simulink model "B2B_2x15kW_LCO_paralelo_y_serie"  (R2026b)
settings: Solver=ode5  StopTime=inf  EnableMultiTasking=on
StopFcn:
  | Modelo_Disable_B2B
undefined symbols (not defined in the file): ALPHA_DC, COS_RO, dataStateMachine, DiscIntNeverNeededParam, dq2abc, EN_G, getNormalizedOffset, I_MAX_G, INV_SIN_RO, KAW_CCG, KAW_DC, KI_CCG, KI_DC, KI_PLLG, KP_CCG, KP_DC, KP_PLLG, L12, LIMIT_SAG_DETECT, magnitude, MIN_VDC_READY, Ncount, NDELAY_SAG_DETECT, PORC_DC_STEADS, SAMPLES_SAG_DETECT, simDCcontCurrent1, simDCcontCurrent2, SN_G, Transformations_blocks, ts, Ts_al, TS_C, TS_PLL, UDC_min_al, UDC_Ref_al, VDC_REF, WN_G
libraries: simulink x15, TriPhaseDriveControl x13, powerlib_extras x2, model_hardware_PM15F80C_rev x2, TriphaseXenomaiTarget x1
(part 3 of 4)

== system B2B_2x15kW_LCO_paralelo_y_serie/VSC1 Controller2/Grid Side Measurements/D-LCO FLL/Sequence Detection/LCO_FLL_3_harm_alfa ==
  note: Para que no se valla a inf
  note: los regresamos
      | a la ganancia
      | original
  note: 1 sobre la ganancia
      | del interarmónico
      | 1/0.05 = 20
  v_in : Inport
  reset_LCO_FLL : Inport  Port=2
  Constant1 : Constant  Value=50
  Demux1 : Demux  Outputs=5
  Demux4 : Demux  Outputs=3
  Discrete-Time Integrator1 : DiscreteIntegrator  gainval=[1 1 1]  ExternalReset=either  InitialCondition=[1 1 10]  SampleTime=TS_PLL  ICPrevOutput=DiscIntNeverNeededParam  ICPrevScaledInput=DiscIntNeverNeededParam
  K gain : Constant  Value=0.1
  LCO_FLL_01 : MATLAB Function  TreatAsAtomicUnit=on
  Mux1 : Mux  Inputs=3
  Mux4 : Mux  Inputs=2
  Mux6 : Mux  Inputs=3
  Saturation2 : Saturate  UpperLimit=10000  LowerLimit=-10000
  Sinch 3 harm paralel : Scope
      settings: TimeSpan=0.1  ActiveDisplayYMinimum=-60  ActiveDisplayYMaximum=80  DataLoggingVariableName=LCO_FLL_graph3_paralelo
  Terminator3 : Terminator
  delta w : Scope
      settings: TimeSpan=20  ActiveDisplayYMinimum=-31  ActiveDisplayYMaximum=-24  DataLoggingVariableName=ScopeData4
  freq : Scope
      settings: TimeSpan=10  ActiveDisplayYMinimum=308  ActiveDisplayYMaximum=322  DataLoggingVariableName=w_LCO2_paralelo
  ki1 : Gain  Gain=2
  ki2 : Gain  Gain=1/(2*pi)
  ki3 : Gain  Gain=1/2
  ki4 : Gain  Gain=1/2
  v_out : Outport
  qv_out : Outport  Port=2
  tag scope: f_alfa_3=global
  wires:
  Discrete-Time Integrator1/1 -> Saturation2/1, Demux4/1
  Saturation2/1 -> Mux6/1
  v_in/1 -> ki1/1
  Constant1/1 -> Mux6/2  "A"
  Mux1/1 -> Discrete-Time Integrator1/1
  reset_LCO_FLL/1 -> Discrete-Time Integrator1/2
  Demux4/3 -> delta w/1, Terminator3/1  "x3 -  delta w"
  Demux4/1 -> ki3/1  "x1 - qv '"
  Demux4/2 -> Mux4/2, ki4/1  "x2 - v '"
  Demux1/1 -> LCO_FLL_01/1(x1)
  Mux6/1 -> Demux1/1
  Demux1/2 -> LCO_FLL_01/2(x2)
  Demux1/3 -> LCO_FLL_01/3(x3)
  Demux1/4 -> LCO_FLL_01/4(A)
  Demux1/5 -> LCO_FLL_01/5(v)
  LCO_FLL_01/1(x1p) -> Mux1/1
  LCO_FLL_01/2(x2p) -> Mux1/2
  LCO_FLL_01/3(x3p) -> Mux1/3
  LCO_FLL_01/4(w) -> ki2/1
  ki2/1 -> [f_alfa_3], freq/1
  Mux4/1 -> Sinch 3 harm paralel/1
  ki4/1 -> v_out/1
  ki3/1 -> qv_out/1
  ki1/1 -> Mux4/1, Mux6/3
  K gain/1 -> LCO_FLL_01/6(k)

== system B2B_2x15kW_LCO_paralelo_y_serie/VSC1 Controller2/Grid Side Measurements/D-LCO FLL/Sequence Detection/LCO_FLL_3_harm_alfa1 ==
  note: Para que no se valla a inf
  note: los regresamos
      | a la ganancia
      | original
  note: 1 sobre la ganancia
      | del interarmónico
      | 1/0.05 = 20
  v_in : Inport
  reset_LCO_FLL : Inport  Port=2
  Constant1 : Constant  Value=50
  Demux1 : Demux  Outputs=5
  Demux4 : Demux  Outputs=3
  Discrete-Time Integrator1 : DiscreteIntegrator  gainval=[1 1 1]  ExternalReset=either  InitialCondition=[1 1 10]  SampleTime=TS_PLL  ICPrevOutput=DiscIntNeverNeededParam  ICPrevScaledInput=DiscIntNeverNeededParam
  K gain : Constant  Value=0.1
  LCO_FLL_01 : MATLAB Function  TreatAsAtomicUnit=on
  Mux1 : Mux  Inputs=3
  Mux4 : Mux  Inputs=2
  Mux6 : Mux  Inputs=3
  Saturation2 : Saturate  UpperLimit=10000  LowerLimit=-10000
  Sinch 3 harm serie : Scope
      settings: TimeSpan=0.1  ActiveDisplayYMinimum=-60  ActiveDisplayYMaximum=80  DataLoggingVariableName=LCO_FLL_graph03_serie
  Terminator3 : Terminator
  delta w : Scope
      settings: TimeSpan=20  ActiveDisplayYMinimum=-31  ActiveDisplayYMaximum=-24  DataLoggingVariableName=ScopeData4
  freq alfa 3 : Scope
      settings: TimeSpan=10  ActiveDisplayYMinimum=529  ActiveDisplayYMaximum=536  DataLoggingVariableName=w_LCO2_serie
  ki1 : Gain  Gain=2
  ki2 : Gain  Gain=1/(2*pi)
  ki3 : Gain  Gain=1/2
  ki4 : Gain  Gain=1/2
  v_out : Outport
  qv_out : Outport  Port=2
  tag scope: f_alfa_3_serie=global
  wires:
  Discrete-Time Integrator1/1 -> Saturation2/1, Demux4/1
  Saturation2/1 -> Mux6/1
  v_in/1 -> ki1/1
  Constant1/1 -> Mux6/2  "A"
  Mux1/1 -> Discrete-Time Integrator1/1
  reset_LCO_FLL/1 -> Discrete-Time Integrator1/2
  Demux4/3 -> delta w/1, Terminator3/1  "x3 -  delta w"
  Demux4/1 -> ki3/1  "x1 - qv '"
  Demux4/2 -> Mux4/2, ki4/1  "x2 - v '"
  Demux1/1 -> LCO_FLL_01/1(x1)
  Mux6/1 -> Demux1/1
  Demux1/2 -> LCO_FLL_01/2(x2)
  Demux1/3 -> LCO_FLL_01/3(x3)
  Demux1/4 -> LCO_FLL_01/4(A)
  Demux1/5 -> LCO_FLL_01/5(v)
  LCO_FLL_01/1(x1p) -> Mux1/1
  LCO_FLL_01/2(x2p) -> Mux1/2
  LCO_FLL_01/3(x3p) -> Mux1/3
  LCO_FLL_01/4(w) -> ki2/1
  ki2/1 -> [f_alfa_3_serie], freq alfa 3/1
  ki1/1 -> Mux4/1, Mux6/3
  ki3/1 -> qv_out/1
  ki4/1 -> v_out/1
  Mux4/1 -> Sinch 3 harm serie/1
  K gain/1 -> LCO_FLL_01/6(k)

== system B2B_2x15kW_LCO_paralelo_y_serie/VSC1 Controller2/Grid Side Measurements/D-LCO FLL/Sequence Detection/LCO_FLL_4_harm_alfa ==
  note: Para que no se valla a inf
  note: los regresamos
      | a la ganancia
      | original
  note: 1 sobre la ganancia
      | del interarmónico
      | 1/0.05 = 20
  v_in : Inport
  reset_LCO_FLL : Inport  Port=2
  Constant1 : Constant  Value=150
  Demux1 : Demux  Outputs=5
  Demux4 : Demux  Outputs=3
  Discrete-Time Integrator1 : DiscreteIntegrator  gainval=[1 1 1]  ExternalReset=either  InitialCondition=[1 1 10]  SampleTime=TS_PLL  ICPrevOutput=DiscIntNeverNeededParam  ICPrevScaledInput=DiscIntNeverNeededParam
  K gain : Constant  Value=0.1
  LCO_FLL_01 : MATLAB Function  TreatAsAtomicUnit=on
  Mux1 : Mux  Inputs=3
  Mux4 : Mux  Inputs=2
  Mux6 : Mux  Inputs=3
  Saturation2 : Saturate  UpperLimit=500  LowerLimit=-500
  Sinch 4 harm paralel : Scope
      settings: TimeSpan=0.1  ActiveDisplayYMinimum=-300  ActiveDisplayYMaximum=300  DataLoggingVariableName=LCO_FLL_graph4_paralelo
  Terminator3 : Terminator
  delta w : Scope
      settings: TimeSpan=20  ActiveDisplayYMinimum=-31  ActiveDisplayYMaximum=-24  DataLoggingVariableName=ScopeData4
  freq : Scope
      settings: TimeSpan=10  ActiveDisplayYMinimum=308  ActiveDisplayYMaximum=322  DataLoggingVariableName=w_LCO3_paralelo
  ki1 : Gain  Gain=5
  ki2 : Gain  Gain=1/(2*pi)
  ki3 : Gain  Gain=1/5
  ki4 : Gain  Gain=1/5
  v_out : Outport
  qv_out : Outport  Port=2
  tag scope: f_alfa_4=global
  wires:
  LCO_FLL_01/4(w) -> ki2/1
  LCO_FLL_01/3(x3p) -> Mux1/3
  LCO_FLL_01/2(x2p) -> Mux1/2
  LCO_FLL_01/1(x1p) -> Mux1/1
  Demux1/5 -> LCO_FLL_01/5(v)
  Demux1/4 -> LCO_FLL_01/4(A)
  Demux1/3 -> LCO_FLL_01/3(x3)
  Demux1/2 -> LCO_FLL_01/2(x2)
  Mux6/1 -> Demux1/1
  Demux1/1 -> LCO_FLL_01/1(x1)
  Demux4/2 -> Mux4/2, ki4/1  "x2 - v '"
  Demux4/1 -> ki3/1  "x1 - qv '"
  Demux4/3 -> Terminator3/1, delta w/1  "x3 -  delta w"
  reset_LCO_FLL/1 -> Discrete-Time Integrator1/2
  Mux1/1 -> Discrete-Time Integrator1/1
  Constant1/1 -> Mux6/2  "A"
  v_in/1 -> ki1/1
  Saturation2/1 -> Mux6/1
  Discrete-Time Integrator1/1 -> Demux4/1, Saturation2/1
  ki2/1 -> [f_alfa_4], freq/1
  Mux4/1 -> Sinch 4 harm paralel/1
  ki3/1 -> qv_out/1
  ki4/1 -> v_out/1
  ki1/1 -> Mux4/1, Mux6/3
  K gain/1 -> LCO_FLL_01/6(k)

== system B2B_2x15kW_LCO_paralelo_y_serie/VSC1 Controller2/Grid Side Measurements/D-LCO FLL/Sequence Detection/LCO_FLL_4_harm_alfa1 ==
  note: Para que no se valla a inf
  note: los regresamos
      | a la ganancia
      | original
  note: 1 sobre la ganancia
      | del interarmónico
      | 1/0.05 = 20
  v_in : Inport
  reset_LCO_FLL : Inport  Port=2
  Constant1 : Constant  Value=150
  Demux1 : Demux  Outputs=5
  Demux4 : Demux  Outputs=3
  Discrete-Time Integrator1 : DiscreteIntegrator  gainval=[1 1 1]  ExternalReset=either  InitialCondition=[1 1 10]  SampleTime=TS_PLL  ICPrevOutput=DiscIntNeverNeededParam  ICPrevScaledInput=DiscIntNeverNeededParam
  K gain : Constant  Value=0.1
  LCO_FLL_01 : MATLAB Function  TreatAsAtomicUnit=on
  Mux1 : Mux  Inputs=3
  Mux4 : Mux  Inputs=2
  Mux6 : Mux  Inputs=3
  Saturation2 : Saturate  UpperLimit=5000  LowerLimit=-5000
  Sinch 4 harm serie : Scope
      settings: TimeSpan=0.1  ActiveDisplayYMinimum=-300  ActiveDisplayYMaximum=300  DataLoggingVariableName=LCO_FLL_graph04_serie
  Terminator3 : Terminator
  delta w : Scope
      settings: TimeSpan=20  ActiveDisplayYMinimum=-31  ActiveDisplayYMaximum=-24  DataLoggingVariableName=ScopeData4
  freq alfa 4 : Scope
      settings: TimeSpan=10  ActiveDisplayYMinimum=308  ActiveDisplayYMaximum=322  DataLoggingVariableName=w_LCO3_serie
  ki1 : Gain  Gain=5
  ki2 : Gain  Gain=1/(2*pi)
  ki3 : Gain  Gain=1/5
  ki4 : Gain  Gain=1/5
  v_out : Outport
  qv_out : Outport  Port=2
  tag scope: f_alfa_4_serie=global
  wires:
  LCO_FLL_01/4(w) -> ki2/1
  LCO_FLL_01/3(x3p) -> Mux1/3
  LCO_FLL_01/2(x2p) -> Mux1/2
  LCO_FLL_01/1(x1p) -> Mux1/1
  Demux1/5 -> LCO_FLL_01/5(v)
  Demux1/4 -> LCO_FLL_01/4(A)
  Demux1/3 -> LCO_FLL_01/3(x3)
  Demux1/2 -> LCO_FLL_01/2(x2)
  Mux6/1 -> Demux1/1
  Demux1/1 -> LCO_FLL_01/1(x1)
  Demux4/2 -> Mux4/2, ki4/1  "x2 - v '"
  Demux4/1 -> ki3/1  "x1 - qv '"
  Demux4/3 -> Terminator3/1, delta w/1  "x3 -  delta w"
  reset_LCO_FLL/1 -> Discrete-Time Integrator1/2
  Mux1/1 -> Discrete-Time Integrator1/1
  Constant1/1 -> Mux6/2  "A"
  v_in/1 -> ki1/1
  Saturation2/1 -> Mux6/1
  Discrete-Time Integrator1/1 -> Demux4/1, Saturation2/1
  ki2/1 -> [f_alfa_4_serie], freq alfa 4/1
  K gain/1 -> LCO_FLL_01/6(k)
  ki1/1 -> Mux4/1, Mux6/3
  ki4/1 -> v_out/1
  ki3/1 -> qv_out/1
  Mux4/1 -> Sinch 4 harm serie/1

== system B2B_2x15kW_LCO_paralelo_y_serie/VSC1 Controller2/Grid Side Measurements/D-LCO FLL/Sequence Detection/LCO_FLL_5_harm_alfa ==
  note: Para que no se valla a inf
  note: los regresamos
      | a la ganancia
      | original
  note: 1 sobre la ganancia
      | del interarmónico
      | 1/0.05 = 20
  v_in : Inport
  reset_LCO_FLL : Inport  Port=2
  Constant1 : Constant  Value=150
  Demux1 : Demux  Outputs=5
  Demux4 : Demux  Outputs=3
  Discrete-Time Integrator1 : DiscreteIntegrator  gainval=[1 1 1]  ExternalReset=either  InitialCondition=[1 1 10]  SampleTime=TS_PLL  ICPrevOutput=DiscIntNeverNeededParam  ICPrevScaledInput=DiscIntNeverNeededParam
  K gain : Constant  Value=0.1
  LCO_FLL_01 : MATLAB Function  TreatAsAtomicUnit=on
  Mux1 : Mux  Inputs=3
  Mux4 : Mux  Inputs=2
  Mux6 : Mux  Inputs=3
  Saturation2 : Saturate  UpperLimit=5000  LowerLimit=-5000
  Sinch 5 harm paralel : Scope
      settings: TimeSpan=0.1  ActiveDisplayYMinimum=-300  ActiveDisplayYMaximum=300  DataLoggingVariableName=LCO_FLL_graph5_paralelo
  Terminator3 : Terminator
  delta w : Scope
      settings: TimeSpan=20  ActiveDisplayYMinimum=-31  ActiveDisplayYMaximum=-24  DataLoggingVariableName=ScopeData4
  freq : Scope
      settings: TimeSpan=10  ActiveDisplayYMinimum=308  ActiveDisplayYMaximum=322  DataLoggingVariableName=w_LCO4_paralelo
  ki1 : Gain  Gain=5
  ki2 : Gain  Gain=1/(2*pi)
  ki3 : Gain  Gain=1/5
  ki4 : Gain  Gain=1/5
  v_out : Outport
  qv_out : Outport  Port=2
  tag scope: f_alfa_5=global
  wires:
  Discrete-Time Integrator1/1 -> Saturation2/1, Demux4/1
  Saturation2/1 -> Mux6/1
  v_in/1 -> ki1/1
  Constant1/1 -> Mux6/2  "A"
  Mux1/1 -> Discrete-Time Integrator1/1
  reset_LCO_FLL/1 -> Discrete-Time Integrator1/2
  Demux4/3 -> delta w/1, Terminator3/1  "x3 -  delta w"
  Demux4/1 -> ki3/1  "x1 - qv '"
  Demux4/2 -> Mux4/2, ki4/1  "x2 - v '"
  Demux1/1 -> LCO_FLL_01/1(x1)
  Mux6/1 -> Demux1/1
  Demux1/2 -> LCO_FLL_01/2(x2)
  Demux1/3 -> LCO_FLL_01/3(x3)
  Demux1/4 -> LCO_FLL_01/4(A)
  Demux1/5 -> LCO_FLL_01/5(v)
  LCO_FLL_01/1(x1p) -> Mux1/1
  LCO_FLL_01/2(x2p) -> Mux1/2
  LCO_FLL_01/3(x3p) -> Mux1/3
  LCO_FLL_01/4(w) -> ki2/1
  ki2/1 -> [f_alfa_5], freq/1
  Mux4/1 -> Sinch 5 harm paralel/1
  ki1/1 -> Mux4/1, Mux6/3
  K gain/1 -> LCO_FLL_01/6(k)
  ki3/1 -> qv_out/1
  ki4/1 -> v_out/1

== system B2B_2x15kW_LCO_paralelo_y_serie/VSC1 Controller2/Grid Side Measurements/D-LCO FLL/Sequence Detection/LCO_FLL_5_harm_alfa1 ==
  note: Para que no se valla a inf
  v_in : Inport
  reset_LCO_FLL : Inport  Port=2
  Constant1 : Constant  Value=158
  Demux1 : Demux  Outputs=5
  Demux4 : Demux  Outputs=3
  Discrete-Time Integrator1 : DiscreteIntegrator  gainval=[1 1 1]  ExternalReset=either  InitialCondition=[1 1 10]  SampleTime=TS_PLL  ICPrevOutput=DiscIntNeverNeededParam  ICPrevScaledInput=DiscIntNeverNeededParam
  K gain : Constant  Value=0.1
  LCO_FLL_01 : MATLAB Function  TreatAsAtomicUnit=on
  Mux1 : Mux  Inputs=3
  Mux6 : Mux  Inputs=3
  Saturation2 : Saturate  UpperLimit=5000  LowerLimit=-5000
  Terminator3 : Terminator
  delta w : Scope
      settings: TimeSpan=20  ActiveDisplayYMinimum=-31  ActiveDisplayYMaximum=-24  DataLoggingVariableName=ScopeData4
  freq alfa 5 : Scope
      settings: TimeSpan=10  ActiveDisplayYMinimum=308  ActiveDisplayYMaximum=322  DataLoggingVariableName=w_LCO4_serie
  ki2 : Gain  Gain=1/(2*pi)
  v_out : Outport
  qv_out : Outport  Port=2
  wires:
  Discrete-Time Integrator1/1 -> Saturation2/1, Demux4/1
  Saturation2/1 -> Mux6/1
  v_in/1 -> Mux6/3
  Constant1/1 -> Mux6/2  "A"
  Mux1/1 -> Discrete-Time Integrator1/1
  reset_LCO_FLL/1 -> Discrete-Time Integrator1/2
  Demux4/3 -> delta w/1, Terminator3/1  "x3 -  delta w"
  Demux4/1 -> qv_out/1  "x1 - qv '"
  Demux4/2 -> v_out/1  "x2 - v '"
  Demux1/1 -> LCO_FLL_01/1(x1)
  Mux6/1 -> Demux1/1
  Demux1/2 -> LCO_FLL_01/2(x2)
  Demux1/3 -> LCO_FLL_01/3(x3)
  Demux1/4 -> LCO_FLL_01/4(A)
  Demux1/5 -> LCO_FLL_01/5(v)
  LCO_FLL_01/1(x1p) -> Mux1/1
  LCO_FLL_01/2(x2p) -> Mux1/2
  LCO_FLL_01/3(x3p) -> Mux1/3
  LCO_FLL_01/4(w) -> ki2/1
  ki2/1 -> freq alfa 5/1
  K gain/1 -> LCO_FLL_01/6(k)

== system B2B_2x15kW_LCO_paralelo_y_serie/VSC1 Controller2/Grid Side Measurements/D-LCO FLL/Sequence Detection/LCO_FLL_main_ALFA ==
  note: Para que no se valla a inf
  note: 1 sobre la ganancia
      | del interarmónico
      | 1/0.05 = 20
  note: los regresamos
      | a la ganancia
      | original
  v_in : Inport
  reset_LCO_FLL : Inport  Port=2
  Constant1 : Constant  Value=158
  Demux1 : Demux  Outputs=5
  Demux4 : Demux  Outputs=3
  Discrete-Time Integrator1 : DiscreteIntegrator  gainval=[1 1 1]  ExternalReset=either  InitialCondition=[1 1 10]  SampleTime=TS_PLL  ICPrevOutput=DiscIntNeverNeededParam  ICPrevScaledInput=DiscIntNeverNeededParam
  K gain : Constant  Value=0.1
  LCO_FLL_01 : MATLAB Function  TreatAsAtomicUnit=on
  Mux1 : Mux  Inputs=3
  Mux4 : Mux  Inputs=2
  Mux6 : Mux  Inputs=3
  Saturation2 : Saturate  UpperLimit=500  LowerLimit=-500
  Sinch 1 harm paralel : Scope
      settings: TimeSpan=0.1  ActiveDisplayYMinimum=-200  ActiveDisplayYMaximum=200  DataLoggingVariableName=LCO_FLL_graph1_paralelo
  Terminator3 : Terminator
  delta w : Scope
      settings: TimeSpan=20  ActiveDisplayYMinimum=-31  ActiveDisplayYMaximum=-24  DataLoggingVariableName=ScopeData4
  freq : Scope
      settings: TimeSpan=10  ActiveDisplayYMinimum=308  ActiveDisplayYMaximum=322  DataLoggingVariableName=w_LCO
  ki1 : Gain
  ki2 : Gain  Gain=1/(2*pi)
  ki3 : Gain
  ki4 : Gain
  v_out : Outport
  qv_out : Outport  Port=2
  tag scope: f_alfa_1=global, w_alfa_LCO=global
  wires:
  Discrete-Time Integrator1/1 -> Saturation2/1, Demux4/1
  Saturation2/1 -> Mux6/1
  v_in/1 -> ki1/1
  Constant1/1 -> Mux6/2  "A"
  Mux1/1 -> Discrete-Time Integrator1/1
  reset_LCO_FLL/1 -> Discrete-Time Integrator1/2
  Demux4/3 -> delta w/1, Terminator3/1  "x3 -  delta w"
  Demux4/1 -> ki3/1  "x1 - qv '"
  Demux4/2 -> Mux4/2, ki4/1  "x2 - v '"
  Demux1/1 -> LCO_FLL_01/1(x1)
  Mux6/1 -> Demux1/1
  Demux1/2 -> LCO_FLL_01/2(x2)
  Demux1/3 -> LCO_FLL_01/3(x3)
  Demux1/4 -> LCO_FLL_01/4(A)
  Demux1/5 -> LCO_FLL_01/5(v)
  LCO_FLL_01/1(x1p) -> Mux1/1
  LCO_FLL_01/2(x2p) -> Mux1/2
  LCO_FLL_01/3(x3p) -> Mux1/3
  LCO_FLL_01/4(w) -> [w_alfa_LCO], ki2/1
  ki2/1 -> [f_alfa_1], freq/1
  ki1/1 -> Mux4/1, Mux6/3
  ki4/1 -> v_out/1
  ki3/1 -> qv_out/1
  K gain/1 -> LCO_FLL_01/6(k)
  Mux4/1 -> Sinch 1 harm paralel/1

== system B2B_2x15kW_LCO_paralelo_y_serie/VSC1 Controller2/Grid Side Measurements/D-LCO FLL/Sequence Detection/LCO_FLL_main_ALFA1 ==
  note: Para que no se valla a inf
  note: 1 sobre la ganancia
      | del interarmónico
      | 1/0.05 = 20
  note: los regresamos
      | a la ganancia
      | original
  v_in : Inport
  reset_LCO_FLL : Inport  Port=2
  Constant1 : Constant  Value=158
  Demux1 : Demux  Outputs=5
  Demux4 : Demux  Outputs=3
  Discrete-Time Integrator1 : DiscreteIntegrator  gainval=[1 1 1]  ExternalReset=either  InitialCondition=[1 1 10]  SampleTime=TS_PLL  ICPrevOutput=DiscIntNeverNeededParam  ICPrevScaledInput=DiscIntNeverNeededParam
  K gain : Constant  Value=0.1
  LCO_FLL_01 : MATLAB Function  TreatAsAtomicUnit=on
  Mux1 : Mux  Inputs=3
  Mux4 : Mux  Inputs=2
  Mux6 : Mux  Inputs=3
  Saturation2 : Saturate  UpperLimit=500  LowerLimit=-500
  Sinch 1 harm serie : Scope
      settings: TimeSpan=0.1  ActiveDisplayYMinimum=-200  ActiveDisplayYMaximum=200  DataLoggingVariableName=LCO_FLL_graph01_serie1
  Terminator3 : Terminator
  delta w : Scope
      settings: TimeSpan=20  ActiveDisplayYMinimum=-31  ActiveDisplayYMaximum=-24  DataLoggingVariableName=ScopeData4
  freq alfa 1 : Scope
      settings: TimeSpan=10  ActiveDisplayYMinimum=0  ActiveDisplayYMaximum=1  DataLoggingVariableName=w_LCO01_serie
  ki1 : Gain
  ki2 : Gain  Gain=1/(2*pi)
  ki3 : Gain
  ki4 : Gain
  v_out : Outport
  qv_out : Outport  Port=2
  tag scope: f_alfa_1_serie=global, w_alfa_LCO_serie=global
  wires:
  Discrete-Time Integrator1/1 -> Saturation2/1, Demux4/1
  Saturation2/1 -> Mux6/1
  v_in/1 -> ki1/1
  Constant1/1 -> Mux6/2  "A"
  Mux1/1 -> Discrete-Time Integrator1/1
  reset_LCO_FLL/1 -> Discrete-Time Integrator1/2
  Demux4/3 -> delta w/1, Terminator3/1  "x3 -  delta w"
  Demux4/1 -> ki3/1  "x1 - qv '"
  Demux4/2 -> Mux4/2, ki4/1  "x2 - v '"
  Demux1/1 -> LCO_FLL_01/1(x1)
  Mux6/1 -> Demux1/1
  Demux1/2 -> LCO_FLL_01/2(x2)
  Demux1/3 -> LCO_FLL_01/3(x3)
  Demux1/4 -> LCO_FLL_01/4(A)
  Demux1/5 -> LCO_FLL_01/5(v)
  LCO_FLL_01/1(x1p) -> Mux1/1
  LCO_FLL_01/2(x2p) -> Mux1/2
  LCO_FLL_01/3(x3p) -> Mux1/3
  LCO_FLL_01/4(w) -> [w_alfa_LCO_serie], ki2/1
  ki2/1 -> [f_alfa_1_serie], freq alfa 1/1
  ki1/1 -> Mux4/1, Mux6/3
  ki4/1 -> v_out/1
  ki3/1 -> qv_out/1
  K gain/1 -> LCO_FLL_01/6(k)
  Mux4/1 -> Sinch 1 harm serie/1

== system B2B_2x15kW_LCO_paralelo_y_serie/VSC1 Controller2/Grid Side Measurements/D-LCO FLL/Sequence Detection/abc to ab ==
  vscG_egabc : Inport
  Fcn5 : Fcn  Expr=sqrt(2/3)*(u[1]-0.5*u[2]-0.5*u[3])
  Fcn6 : Fcn  Expr=sqrt(1/2)*(u[2]-u[3])
  Mux4 : Mux  Inputs=2
  ki1 : Gain  Gain=sqrt(2/3)
  out : Outport
  wires:
  vscG_egabc/1 -> Fcn5/1, Fcn6/1
  Fcn5/1 -> Mux4/1
  Fcn6/1 -> Mux4/2
  Mux4/1 -> ki1/1
  ki1/1 -> out/1

== system B2B_2x15kW_LCO_paralelo_y_serie/VSC2 Controller/Grid Side Measurements/DSOGI QSG PLL/Sequence Detection/SOGI a  ==
  in : Inport
  w : Inport  Port=2
  Add1 : Sum  Inputs=|+-
  Add2 : Sum  Inputs=|++
  Add3 : Sum  Inputs=|++
  Product1 : Product  RndMeth=Zero
  Product3 : Product  RndMeth=Zero
  Product6 : Product  RndMeth=Zero
  STEP_Q23 : Constant  Value=TS_PLL  SampleTime=TS_PLL
  Unit Delay : UnitDelay  SampleTime=-1
  Unit Delay1 : UnitDelay  SampleTime=-1
  Unit Delay2 : UnitDelay  SampleTime=-1
  v' : Outport
  qv' : Outport  Port=2
  wires:
  Product6/1 -> Product1/1, Product3/2  "step_w"
  STEP_Q23/1 -> Product6/1
  Product1/1 -> Add3/1  "pre_qalpha"
  w/1 -> Product6/2
  in/1 -> Add1/1
  Add1/1 -> Product3/1  "error_qalfa"
  Product3/1 -> Add2/1  "prealfa"
  Add2/1 -> v'/1, Product1/2, Unit Delay/1  "alpha"
  Add3/1 -> qv'/1, Unit Delay2/1, Unit Delay1/1
  Unit Delay2/1 -> Add3/2
  Unit Delay/1 -> Add2/2
  Unit Delay1/1 -> Add1/2

== system B2B_2x15kW_LCO_paralelo_y_serie/VSC2 Controller/Grid Side Measurements/DSOGI QSG PLL/Sequence Detection/SOGI b ==
  in : Inport
  w : Inport  Port=2
  Add1 : Sum  Inputs=|+-
  Add2 : Sum  Inputs=|++
  Add3 : Sum  Inputs=|++
  Product1 : Product  RndMeth=Zero
  Product3 : Product  RndMeth=Zero
  Product6 : Product  RndMeth=Zero
  STEP_Q23 : Constant  Value=TS_PLL  SampleTime=TS_PLL
  Unit Delay1 : UnitDelay  SampleTime=-1
  Unit Delay2 : UnitDelay  SampleTime=-1
  Unit Delay3 : UnitDelay  SampleTime=-1
  v' : Outport
  qv' : Outport  Port=2
  wires:
  Unit Delay3/1 -> Add1/2
  Unit Delay1/1 -> Add2/2
  Unit Delay2/1 -> Add3/2
  Add3/1 -> qv'/1, Unit Delay2/1, Unit Delay3/1
  Add2/1 -> Product1/2, v'/1, Unit Delay1/1  "alpha"
  Product3/1 -> Add2/1  "prealpha"
  Add1/1 -> Product3/1  "error_qalfa"
  in/1 -> Add1/1
  w/1 -> Product6/2
  Product1/1 -> Add3/1  "pre_qalpha"
  STEP_Q23/1 -> Product6/1
  Product6/1 -> Product3/2, Product1/1  "step_w"

== system B2B_2x15kW_LCO_paralelo_y_serie/VSC2 Controller/Grid Side Measurements/DSOGI QSG PLL/Sequence Detection/abc to ab ==
  vscG_egabc : Inport
  Fcn5 : Fcn  Expr=sqrt(2/3)*(u[1]-0.5*u[2]-0.5*u[3])
  Fcn6 : Fcn  Expr=sqrt(1/2)*(u[2]-u[3])
  Mux4 : Mux  Inputs=2
  ki1 : Gain  Gain=sqrt(2/3)
  out : Outport
  wires:
  vscG_egabc/1 -> Fcn5/1, Fcn6/1
  Fcn5/1 -> Mux4/1
  Fcn6/1 -> Mux4/2
  Mux4/1 -> ki1/1
  ki1/1 -> out/1

== matlab function B2B_2x15kW_LCO_paralelo_y_serie/VSC2 Controller/dq to abc/udq Limitation ==
  settings: fimath=|
      | fimath(...
      | 'RoundMode', 'floor',...
      | 'OverflowMode', 'wrap',...
      | 'ProductMode', 'KeepLSB', 'ProductWordLength', 32,...
      | 'SumMode', 'KeepLSB', 'SumWordLength', 32,...
      | 'CastBeforeSum', false)
  data: vscG_ugdqRef input size=2; vscG_egdqPos input; vscG_ugdqSat output size=2; WNG_L12_IMAXG input
%Name: Saturation of the reference voltage inside the unit circle
%Developed: Emilio Bueno
%Modified: Javier Roldan

function vscG_ugdqSat = fcn(vscG_ugdqRef, vscG_egdqPos, WNG_L12_IMAXG)

%Definition of the inputs
ud_c = vscG_ugdqRef(1);
uq_c = vscG_ugdqRef(2);
WN_G = WNG_L12_IMAXG(1);
L12 = WNG_L12_IMAXG(2);
I_MAX_G = WNG_L12_IMAXG(3);

%Initialisation of the outputs
vscG_ugdqSat = [0 0]';

%We obtain the modulus
edq = sqrt(vscG_egdqPos(1)^2+vscG_egdqPos(2)^2)*(sqrt(2/3)); %Invariant power transformation, sqrt(2/3)

%Calculation of the maximum values
I_MAX_G_PEAK = I_MAX_G*sqrt(2);          %Maximum peak value
udqmax       = edq+WN_G*L12*I_MAX_G_PEAK;  %Maximum reachable voltage
udqmin       = edq-WN_G*L12*I_MAX_G_PEAK;  %Minimum reachable voltage

%We obtain the angle
theta = atan2(uq_c, ud_c);

%Saturation of the output
if ((ud_c*ud_c)+(uq_c*uq_c)) > (udqmax*udqmax*sqrt(2)) %Ouside the circle
    %vscG_ugdqSat(1) = udqmax*cos(theta);
    %vscG_ugdqSat(2) = udqmax*sin(theta); 
    vscG_ugdqSat(1) = ud_c;
    vscG_ugdqSat(2) = uq_c;
elseif ((ud_c*ud_c)+(uq_c*uq_c)) < (udqmin*udqmin*sqrt(2)) %Outside the circle
    %vscG_ugdqSat(1) = udqmin*cos(theta); 
    %vscG_ugdqSat(2) = udqmin*sin(theta);
    vscG_ugdqSat(1) = ud_c;
    vscG_ugdqSat(2) = uq_c;
else    %With no constraint
    vscG_ugdqSat(1) = ud_c;
    vscG_ugdqSat(2) = uq_c;
end

== matlab function B2B_2x15kW_LCO_paralelo_y_serie/VSC1 Controller2/Grid Side Measurements/D-LCO FLL/Sequence Detection/LCO_FLL_main_ALFA/LCO_FLL_01 ==
  settings: fimath=|
      | fimath(...
      | 'RoundMode', 'floor',...
      | 'OverflowMode', 'wrap',...
      | 'ProductMode', 'KeepLSB', 'ProductWordLength', 32,...
      | 'SumMode', 'KeepLSB', 'SumWordLength', 32,...
      | 'CastBeforeSum', false)
  data: x1 input; x1p output; x2 input; x3 input; A input; v input; x2p output; x3p output; w output; k input
function [x1p,x2p,x3p,w] = fcn(x1, x2, x3, A, v, k)

%16/11/2021
%LCO-FLL for around 50Hz
%By Erick Israel Vázquez Oviedo
% Constants
wffw = 2*pi*55; %Initial frequency 
% k = 2; a controlar
gama = 1;
w = x3 + wffw;
ev = v - x2; % Error between reference and x2 to synchronize

% Diferential equations
x1p = (           (x1) + (x2) - ((1/(A*A))*x1*((x1*x1)+(x2*x2)))  )*w;
x2p = ( (k*ev) + (-x1) + (x2) - ((1/(A*A))*x2*((x1*x1)+(x2*x2)))  )*w;
x3p = -gama*ev*x1; % x1 is in quadrature with x2, 90 degrees delay

== matlab function B2B_2x15kW_LCO_paralelo_y_serie/VSC1 Controller2/Grid Side Measurements/D-LCO FLL/Sequence Detection/LCO_FLL_4_harm_alfa/LCO_FLL_01 ==
  settings: fimath=|
      | fimath(...
      | 'RoundMode', 'floor',...
      | 'OverflowMode', 'wrap',...
      | 'ProductMode', 'KeepLSB', 'ProductWordLength', 32,...
      | 'SumMode', 'KeepLSB', 'SumWordLength', 32,...
      | 'CastBeforeSum', false)
  data: x1 input; x1p output; x2 input; x3 input; A input; v input; x2p output; x3p output; w output; k input
function [x1p,x2p,x3p,w] = fcn(x1, x2, x3, A, v, k)

%16/11/2021
%LCO-FLL for around 50Hz
%By Erick Israel Vázquez Oviedo
% Constants
wffw = 2*pi*850; %Initial frequency 
%k = 2; a controlar
gama = 1;
w = x3 + wffw;
ev = v - x2; % Error between reference and x2 to synchronize

% Diferential equations
x1p = (           (x1) + (x2) - ((1/(A*A))*x1*((x1*x1)+(x2*x2)))  )*w;
x2p = ( (k*ev) + (-x1) + (x2) - ((1/(A*A))*x2*((x1*x1)+(x2*x2)))  )*w;
x3p = -gama*ev*x1; % x1 is in quadrature with x2, 90 degrees delay

== matlab function B2B_2x15kW_LCO_paralelo_y_serie/VSC1 Controller2/Grid Side Measurements/D-LCO FLL/Sequence Detection/LCO_FLL_5_harm_alfa/LCO_FLL_01 ==
  settings: fimath=|
      | fimath(...
      | 'RoundMode', 'floor',...
      | 'OverflowMode', 'wrap',...
      | 'ProductMode', 'KeepLSB', 'ProductWordLength', 32,...
      | 'SumMode', 'KeepLSB', 'SumWordLength', 32,...
      | 'CastBeforeSum', false)
  data: x1 input; x1p output; x2 input; x3 input; A input; v input; x2p output; x3p output; w output; k input
function [x1p,x2p,x3p,w] = fcn(x1, x2, x3, A, v, k)

%16/11/2021
%LCO-FLL for around 50Hz
%By Erick Israel Vázquez Oviedo
% Constants
wffw = 2*pi*850; %Initial frequency 
%k = 2; a controlar
gama = 1;
w = x3 + wffw;
ev = v - x2; % Error between reference and x2 to synchronize

% Diferential equations
x1p = (           (x1) + (x2) - ((1/(A*A))*x1*((x1*x1)+(x2*x2)))  )*w;
x2p = ( (k*ev) + (-x1) + (x2) - ((1/(A*A))*x2*((x1*x1)+(x2*x2)))  )*w;
x3p = -gama*ev*x1; % x1 is in quadrature with x2, 90 degrees delay

== matlab function B2B_2x15kW_LCO_paralelo_y_serie/VSC1 Controller2/Grid Side Measurements/D-LCO FLL/Sequence Detection/LCO_FLL_3_harm_alfa1/LCO_FLL_01 ==
  settings: fimath=|
      | fimath(...
      | 'RoundMode', 'floor',...
      | 'OverflowMode', 'wrap',...
      | 'ProductMode', 'KeepLSB', 'ProductWordLength', 32,...
      | 'SumMode', 'KeepLSB', 'SumWordLength', 32,...
      | 'CastBeforeSum', false)
  data: x1 input; x1p output; x2 input; x3 input; A input; v input; x2p output; x3p output; w output; k input
function [x1p,x2p,x3p,w] = fcn(x1, x2, x3, A, v, k)

%16/11/2021
%LCO-FLL for around 50Hz
%By Erick Israel Vázquez Oviedo
% Constants
wffw = 2*pi*550; %Initial frequency 
%k = 0.1; a controlar
gama = 1;
w = x3 + wffw;
ev = v - x2; % Error between reference and x2 to synchronize

% Diferential equations
x1p = (           (x1) + (x2) - ((1/(A*A))*x1*((x1*x1)+(x2*x2)))  )*w;
x2p = ( (k*ev) + (-x1) + (x2) - ((1/(A*A))*x2*((x1*x1)+(x2*x2)))  )*w;
x3p = -gama*ev*x1; % x1 is in quadrature with x2, 90 degrees delay

== matlab function B2B_2x15kW_LCO_paralelo_y_serie/VSC1 Controller2/Grid Side Measurements/D-LCO FLL/Sequence Detection/LCO_FLL_4_harm_alfa1/LCO_FLL_01 ==
  settings: fimath=|
      | fimath(...
      | 'RoundMode', 'floor',...
      | 'OverflowMode', 'wrap',...
      | 'ProductMode', 'KeepLSB', 'ProductWordLength', 32,...
      | 'SumMode', 'KeepLSB', 'SumWordLength', 32,...
      | 'CastBeforeSum', false)
  data: x1 input; x1p output; x2 input; x3 input; A input; v input; x2p output; x3p output; w output; k input
function [x1p,x2p,x3p,w] = fcn(x1, x2, x3, A, v, k)

%16/11/2021
%LCO-FLL for around 50Hz
%By Erick Israel Vázquez Oviedo
% Constants
wffw = 2*pi*850; %Initial frequency 
%k = 0.1; a controlar
gama = 1;
w = x3 + wffw;
ev = v - x2; % Error between reference and x2 to synchronize

% Diferential equations
x1p = (           (x1) + (x2) - ((1/(A*A))*x1*((x1*x1)+(x2*x2)))  )*w;
x2p = ( (k*ev) + (-x1) + (x2) - ((1/(A*A))*x2*((x1*x1)+(x2*x2)))  )*w;
x3p = -gama*ev*x1; % x1 is in quadrature with x2, 90 degrees delay

== matlab function B2B_2x15kW_LCO_paralelo_y_serie/VSC1 Controller2/Grid Side Measurements/D-LCO FLL/Sequence Detection/LCO_FLL_5_harm_alfa1/LCO_FLL_01 ==
  settings: fimath=|
      | fimath(...
      | 'RoundMode', 'floor',...
      | 'OverflowMode', 'wrap',...
      | 'ProductMode', 'KeepLSB', 'ProductWordLength', 32,...
      | 'SumMode', 'KeepLSB', 'SumWordLength', 32,...
      | 'CastBeforeSum', false)
  data: x1 input; x1p output; x2 input; x3 input; A input; v input; x2p output; x3p output; w output; k input
function [x1p,x2p,x3p,w] = fcn(x1, x2, x3, A, v, k)

%16/11/2021
%LCO-FLL for around 50Hz
%By Erick Israel Vázquez Oviedo
% Constants
wffw = 2*pi*550; %Initial frequency 
%k = 0.1; a controlar
gama = 1;
w = x3 + wffw;
ev = v - x2; % Error between reference and x2 to synchronize

% Diferential equations
x1p = (           (x1) + (x2) - ((1/(A*A))*x1*((x1*x1)+(x2*x2)))  )*w;
x2p = ( (k*ev) + (-x1) + (x2) - ((1/(A*A))*x2*((x1*x1)+(x2*x2)))  )*w;
x3p = -gama*ev*x1; % x1 is in quadrature with x2, 90 degrees delay

== matlab function B2B_2x15kW_LCO_paralelo_y_serie/VSC1 Controller2/DC link Voltage Controller/Grid Current Reference Calculation ==
  settings: fimath=|
      | fimath(...
      | 'RoundMode', 'floor',...
      | 'OverflowMode', 'wrap',...
      | 'ProductMode', 'KeepLSB', 'ProductWordLength', 32,...
      | 'SumMode', 'KeepLSB', 'SumWordLength', 32,...
      | 'CastBeforeSum', false)
  data: vscG_qgRef input; vscG_pgRef input; vscG_i2dqRef output size=2; Pg output; vscG_egdqPos input size=2; SNG_IMAXG input
function [vscG_i2dqRef, Pg] = fcn(vscG_qgRef, vscG_pgRef, vscG_egdqPos, SNG_IMAXG)

%Initialisation of the outputs
vscG_i2dqRef = [0 0]';

%Definition of the inputs
Pgref = vscG_pgRef;             %Active power before saturation
Qgref = vscG_qgRef;             %Reactive power before saturation
edp = vscG_egdqPos(1);          %d-axis component of the grid voltage positive sequence
eqp = vscG_egdqPos(2);          %q-axis component of the grid voltage positive sequence
SN_G = SNG_IMAXG(1);    %Nominal aparent power (20% larger than nominal for transients)
I_MAX_G = SNG_IMAXG(2); %Nominal grid current

%Limitation of active power
Pgmax = SN_G;
if (Pgref > Pgmax) 
    Pg = Pgmax;
elseif (Pgref < -Pgmax)  
    Pg = -Pgmax;
else
    Pg = Pgref; 
end

%Limitation of reactive power
Qgmax = sqrt(SN_G^2-Pg^2);     %To have some degree of regulation
if (Qgref > Qgmax) 
    Qg = Qgmax;
elseif (Qgref < -Qgmax)  
    Qg = -Qgmax;
else
    Qg = Qgref; 
end

%Limitation of d-axis (active) current
%idref = Pg/(sqrt(edp^2+eqp^2)+eps)*2/3;
idref = (Pg*edp+Qg*eqp)/(edp^2+eqp^2+eps);
idref = idref*2/3;
if (idref > I_MAX_G) 
    id = I_MAX_G;
elseif (idref < -I_MAX_G)  
    id = -I_MAX_G;
else
    id = idref;
end

%Limtiation of q-axis (reactive) current
%iqref = -Qg/(sqrt(edp^2+eqp^2)+eps)*2/3;
iqref = (+Pg*eqp-Qg*edp)/(edp^2+eqp^2+eps);
iqref = iqref*2/3;
iqrefmax = sqrt(I_MAX_G^2-id^2);
if (iqref > iqrefmax) 
    iq = iqrefmax;
elseif (iqref < -iqrefmax)  
    iq = -iqrefmax;
else
    iq = iqref;
end

%Definition of the outputs
vscG_i2dqRef(1) = id;
vscG_i2dqRef(2) = iq;

== matlab function B2B_2x15kW_LCO_paralelo_y_serie/VSC1 Controller2/Grid Side Measurements/D-LCO FLL/Sequence Detection/LCO_FLL_main_ALFA1/LCO_FLL_01 ==
  settings: fimath=|
      | fimath(...
      | 'RoundMode', 'floor',...
      | 'OverflowMode', 'wrap',...
      | 'ProductMode', 'KeepLSB', 'ProductWordLength', 32,...
      | 'SumMode', 'KeepLSB', 'SumWordLength', 32,...
      | 'CastBeforeSum', false)
  data: x1 input; x1p output; x2 input; x3 input; A input; v input; x2p output; x3p output; w output; k input
function [x1p,x2p,x3p,w] = fcn(x1, x2, x3, A, v, k)

%16/11/2021
%LCO-FLL for around 50Hz
%By Erick Israel Vázquez Oviedo
% Constants
wffw = 2*pi*55; %Initial frequency 
%k = 0.1; a controlar
gama = 1;
w = x3 + wffw;
ev = v - x2; % Error between reference and x2 to synchronize

% Diferential equations
x1p = (           (x1) + (x2) - ((1/(A*A))*x1*((x1*x1)+(x2*x2)))  )*w;
x2p = ( (k*ev) + (-x1) + (x2) - ((1/(A*A))*x2*((x1*x1)+(x2*x2)))  )*w;
x3p = -gama*ev*x1; % x1 is in quadrature with x2, 90 degrees delay

== matlab function B2B_2x15kW_LCO_paralelo_y_serie/VSC2 Controller/DC link Voltage Controller/Grid Current Reference Calculation ==
  settings: fimath=|
      | fimath(...
      | 'RoundMode', 'floor',...
      | 'OverflowMode', 'wrap',...
      | 'ProductMode', 'KeepLSB', 'ProductWordLength', 32,...
      | 'SumMode', 'KeepLSB', 'SumWordLength', 32,...
      | 'CastBeforeSum', false)
  data: vscG_qgRef input; vscG_pgRef input; vscG_i2dqRef output size=2; Pg output; vscG_egdqPos input size=2; SNG_IMAXG input
function [vscG_i2dqRef, Pg] = fcn(vscG_qgRef, vscG_pgRef, vscG_egdqPos, SNG_IMAXG)

%Initialisation of the outputs
vscG_i2dqRef = [0 0]';

%Definition of the inputs
Pgref = vscG_pgRef;             %Active power before saturation
Qgref = vscG_qgRef;             %Reactive power before saturation
edp = vscG_egdqPos(1);          %d-axis component of the grid voltage positive sequence
eqp = vscG_egdqPos(2);          %q-axis component of the grid voltage positive sequence
SN_G = SNG_IMAXG(1);    %Nominal aparent power (20% larger than nominal for transients)
I_MAX_G = SNG_IMAXG(2); %Nominal grid current

%Limitation of active power
Pgmax = SN_G;
if (Pgref > Pgmax) 
    Pg = Pgmax;
elseif (Pgref < -Pgmax)  
    Pg = -Pgmax;
else
    Pg = Pgref; 
end

%Limitation of reactive power
Qgmax = sqrt(SN_G^2-Pg^2);     %To have some degree of regulation
if (Qgref > Qgmax) 
    Qg = Qgmax;
elseif (Qgref < -Qgmax)  
    Qg = -Qgmax;
else
    Qg = Qgref; 
end

%Limitation of d-axis (active) current
%idref = Pg/(sqrt(edp^2+eqp^2)+eps)*2/3;
idref = (Pg*edp+Qg*eqp)/(edp^2+eqp^2+eps);
idref = idref*2/3;
if (idref > I_MAX_G) 
    id = I_MAX_G;
elseif (idref < -I_MAX_G)  
    id = -I_MAX_G;
else
    id = idref;
end

%Limtiation of q-axis (reactive) current
%iqref = -Qg/(sqrt(edp^2+eqp^2)+eps)*2/3;
iqref = (+Pg*eqp-Qg*edp)/(edp^2+eqp^2+eps);
iqref = iqref*2/3;
iqrefmax = sqrt(I_MAX_G^2-id^2);
if (iqref > iqrefmax) 
    iq = iqrefmax;
elseif (iqref < -iqrefmax)  
    iq = -iqrefmax;
else
    iq = iqref;
end

%Definition of the outputs
vscG_i2dqRef(1) = id;
vscG_i2dqRef(2) = iq;

== matlab function B2B_2x15kW_LCO_paralelo_y_serie/VSC1 Controller2/Grid Side Measurements/D-LCO FLL/Sequence Detection/Sequence Detection ==
  settings: fimath=|
      | fimath(...
      | 'RoundMode', 'floor',...
      | 'OverflowMode', 'wrap',...
      | 'ProductMode', 'KeepLSB', 'ProductWordLength', 32,...
      | 'SumMode', 'KeepLSB', 'SumWordLength', 32,...
      | 'CastBeforeSum', false)
  data: ealphapos input; input_pll output; secuencia output; ebetapos input; ealphaneg input; ebetaneg input; theta input; edpos output; eqpos output; edneg output; eqneg output
function [input_pll, secuencia, edpos, eqpos, edneg, eqneg] = fcn(ealphapos, ebetapos, ealphaneg, ebetaneg, theta)

%Computation of negative and positive sequence module
module_ealphabetapos = sqrt(ealphapos^2+ebetapos^2);
module_ealphabetaneg = sqrt(ealphaneg^2+ebetaneg^2);

%Sequence detection
if (module_ealphabetapos >= module_ealphabetaneg)
    secuencia = +1; %Positive sequence
else
    secuencia = -1; %Negative sequence
end

%Positive sequence calculation
edpos = ealphapos*cos(theta)+ebetapos*sin(theta);
eqpos = -ealphapos*sin(theta)+ebetapos*cos(theta);

%Negative sequence calculation
edneg = ealphaneg*cos(theta)-ebetaneg*sin(theta);
eqneg = ealphaneg*sin(theta)+ebetaneg*cos(theta);

%Output calculation
if (secuencia == 1)
    eqpos_pu = eqpos/module_ealphabetapos;
    input_pll = eqpos_pu;
else 
    eqneg_pu = eqneg/module_ealphabetaneg;
    input_pll = eqneg_pu;
end

== matlab function B2B_2x15kW_LCO_paralelo_y_serie/VSC1 Controller2/State Machine/State Machine ==
  settings: fimath=|
      | fimath(...
      | 'RoundMode', 'floor',...
      | 'OverflowMode', 'wrap',...
      | 'ProductMode', 'KeepLSB', 'ProductWordLength', 32,...
      | 'SumMode', 'KeepLSB', 'SumWordLength', 32,...
      | 'CastBeforeSum', false)
  data: data input; outputs output; nowState output; nowCounters output; inputs input size=6; prevState input; prevCounters input
function [outputs, nowState, nowCounters] = fcn(data, inputs, prevState, prevCounters)

%%%%%%%%%%%%%%%%%%%%%%%%%%%%%%%%%%%%%%%%%%%%%%%%%%%%%%%%%%%%%%%%%%%%%%%%%%%
%List of states
%%%%%%%%%%%%%%%%%%%%%%%%%%%%%%%%%%%%%%%%%%%%%%%%%%%%%%%%%%%%%%%%%%%%%%%%%%%

%1: POWER_ON              : Power on, everything deactivated
%2: PRECHARGE             : Precharge of the DC-link capacitors
%3: STANDBY               : Waiting to start
%4: START                 : Start sequence 
%5: OPERATING             : Normal operation 

%Initial value
state = prevState;

%%%%%%%%%%%%%%%%%%%%%%%%%%%%%%%%%%%%%%%%%%%%%%%%%%%%%%%%%%%%%%%%%%%%%%%%%%%
%List of data
%%%%%%%%%%%%%%%%%%%%%%%%%%%%%%%%%%%%%%%%%%%%%%%%%%%%%%%%%%%%%%%%%%%%%%%%%%%

%1: Nprecharge
%2: Nconnect
%3: NinitCCG

%Set the data to variables
Nprecharge   = data(1);
Nconnect     = data(2);
NinitCCG     = data(3);

%%%%%%%%%%%%%%%%%%%%%%%%%%%%%%%%%%%%%%%%%%%%%%%%%%%%%%%%%%%%%%%%%%%%%%%%%%%
%List of Inputs
%%%%%%%%%%%%%%%%%%%%%%%%%%%%%%%%%%%%%%%%%%%%%%%%%%%%%%%%%%%%%%%%%%%%%%%%%%%

%1:  PRECHARGE         : 0 NO precharge required
%                      : 1 
%2:  CONNECT           : 0 NO connection required
%                      : 1
%3:  SEL_QVCONTROL     : 0 V controller
%                      : 1 Q controller
%4:  VDC_READY         : 0 VDV >= than stablished value
%                      : 1 
%5:  VDC_STEADS        : 0 Not reached DC steady-state
%                      : 1 
%6:  FLAG_SAG          : 0 No voltage sag detected
%                      : 1 

%Set the variables to its names
PRECHARGE     = inputs(1);
CONNECT       = inputs(2);
SEL_QVCONTROL = inputs(3);
VDC_READY     = inputs(4);
VDC_STEADS    = inputs(5);
FLAG_SAG      = inputs(6);

%%%%%%%%%%%%%%%%%%%%%%%%%%%%%%%%%%%%%%%%%%%%%%%%%%%%%%%%%%%%%%%%%%%%%%%%%%%
%List of outputs
%%%%%%%%%%%%%%%%%%%%%%%%%%%%%%%%%%%%%%%%%%%%%%%%%%%%%%%%%%%%%%%%%%%%%%%%%%%

%PWMOnGrid                     : 0 Do NOT PWM of grid converter
%                              : 1 
%CONNECT_GRID_CONTACT          : 0 NO connection to grid
%                              : 1
%CONNECT_PRELOAD_CONTACT       : 0 NO connection of precharge
%                              : 1 
%selReactiveVoltageController  : 0 Selection of V control
%                              : 1 Selection of Q control
%initPLLGrid                   : 0 Do NOT activate the PLL
%                              : 1 
%initReactiveVoltageController : 0 NO activate the external AC control (Q/VAC)
%                              : 1
%initCurrentControllerG        : 0 Do NOT initilialise the current controller
%                              : 1 
%initDCControllerGrid          : 0 Do NOT initialise the DC controller
%                              : 1                        

%Initilisation
PWMOnGrid               = 0;
CONNECT_GRID_CONTACT    = 0;
CONNECT_PRELOAD_CONTACT = 0;
selReactiveVoltageController  = SEL_QVCONTROL;
initPLLGrid             = 0;
initReactiveVoltageController = 0;
initCurrentControllerG  = 0;
initDCControllerGrid    = 0;

%%%%%%%%%%%%%%%%%%%%%%%%%%%%%%%%%%%%%%%%%%%%%%%%%%%%%%%%%%%%%%%%%%%%%%%%%%%
%List of counters
%%%%%%%%%%%%%%%%%%%%%%%%%%%%%%%%%%%%%%%%%%%%%%%%%%%%%%%%%%%%%%%%%%%%%%%%%%%

%Initilisation
CONT_PRECHARGE   = 0;
CONT_CONNECT     = 0;
CONT_INIT_CC     = 0;

%Adjustment of vector counters
CONT_PRECHARGE_ANT   = prevCounters(1);
CONT_CONNECT_ANT     = prevCounters(2);
CONT_INIT_CC_ANT     = prevCounters(3);

%%%%%%%%%%%%%%%%%%%%%%%%%%%%%%%%%%%%%%%%%%%%%%%%%%%%%%%%%%%%%%%%%%%%%%%%%%%
%STATE MACHINE: MAIN SWITCH
%%%%%%%%%%%%%%%%%%%%%%%%%%%%%%%%%%%%%%%%%%%%%%%%%%%%%%%%%%%%%%%%%%%%%%%%%%%

switch prevState

%%%%%%%%%%%%%%%%%%%%%%%%%%%%%%%%%%%%%%%%%%%%%%%%%%%%%%%%%%%%%%%%%%%%%%%%%%%
%STATE 1: POWER_ON
%%%%%%%%%%%%%%%%%%%%%%%%%%%%%%%%%%%%%%%%%%%%%%%%%%%%%%%%%%%%%%%%%%%%%%%%%%%

case 1

%Outputs for the state
PWMOnGrid               = 0;
CONNECT_GRID_CONTACT    = 0;
CONNECT_PRELOAD_CONTACT = 0;
selReactiveVoltageController  = SEL_QVCONTROL;
initPLLGrid             = 0;
initReactiveVoltageController = 0;
initDCControllerGrid    = 0;

%Counter initialisation
CONT_PRECHARGE   = 0;
CONT_CONNECT     = 0;
CONT_INIT_CC     = 0;

%Conditions to change state
if (PRECHARGE == 1) %Precharge
    state = 2;                            %Change to state 2 
end

%%%%%%%%%%%%%%%%%%%%%%%%%%%%%%%%%%%%%%%%%%%%%%%%%%%%%%%%%%%%%%%%%%%%%%%%%%%
%STATE 2: PRECHARGE
%%%%%%%%%%%%%%%%%%%%%%%%%%%%%%%%%%%%%%%%%%%%%%%%%%%%%%%%%%%%%%%%%%%%%%%%%%%

case 2

%Outputs for the state
PWMOnGrid               = 0;
CONNECT_GRID_CONTACT    = 0;
CONNECT_PRELOAD_CONTACT = 1;
selReactiveVoltageController = SEL_QVCONTROL;
initPLLGrid             = 1;
initReactiveVoltageController = 0;
initCurrentControllerG  = 0;
initDCControllerGrid    = 0;

%Counter initialisation
CONT_PRECHARGE   = 1;
CONT_CONNECT     = 0;
CONT_INIT_CC     = 0;

%Conditions to change state
if (PRECHARGE == 0) %If precharge is zero, go init
    state = 1;
end

if ((CONT_PRECHARGE_ANT >= Nprecharge) && (VDC_READY == 1)) % If time for precharge is reached
    state = 3;              %Go to standby
    CONT_PRECHARGE_ANT = 0; %Unload the counter
end

%%%%%%%%%%%%%%%%%%%%%%%%%%%%%%%%%%%%%%%%%%%%%%%%%%%%%%%%%%%%%%%%%%%%%%%%%%%
%STATE 3: STANDBY
%%%%%%%%%%%%%%%%%%%%%%%%%%%%%%%%%%%%%%%%%%%%%%%%%%%%%%%%%%%%%%%%%%%%%%%%%%%

case 3

%Outputs for the state
PWMOnGrid               = 0;
CONNECT_GRID_CONTACT    = 1;
CONNECT_PRELOAD_CONTACT = 0;
selReactiveVoltageController = SEL_QVCONTROL;
initPLLGrid             = 1;
initReactiveVoltageController = 0;
initCurrentControllerG  = 0;
initDCControllerGrid    = 0;

%Counter initialisation
CONT_PRECHARGE   = 0;
CONT_CONNECT     = 1;
CONT_INIT_CC     = 0;

%Conditions to change state
if ((CONT_CONNECT_ANT >= Nconnect) && (CONNECT == 1) && (VDC_STEADS == 1)) %If time to connect is reached
	state = 4; 
    CONT_CONNECT_ANT = 0; %Unload the counter
end

%%%%%%%%%%%%%%%%%%%%%%%%%%%%%%%%%%%%%%%%%%%%%%%%%%%%%%%%%%%%%%%%%%%%%%%%%%%
%STATE 4: START
%%%%%%%%%%%%%%%%%%%%%%%%%%%%%%%%%%%%%%%%%%%%%%%%%%%%%%%%%%%%%%%%%%%%%%%%%%%

case 4

%Outputs for the state
PWMOnGrid               = 1;
CONNECT_GRID_CONTACT    = 1;
CONNECT_PRELOAD_CONTACT = 0;
selReactiveVoltageController = SEL_QVCONTROL;
initPLLGrid             = 1;
initReactiveVoltageController = 0;
initCurrentControllerG  = 1;
initDCControllerGrid    = 1;

%Counter initialisation
CONT_PRECHARGE   = 0;
CONT_CONNECT     = 0;
CONT_INIT_CC     = 1;

%Conditions to change state
if (CONT_INIT_CC_ANT >= NinitCCG)  %If time to start is reached
    state = 5;                     %Go to regular operation
    CONT_INIT_CC_ANT = 0;          %Unload the counter
end

if (CONNECT == 0)  %If connect equals zero
    state = 1;     %Dischonnect
end

%%%%%%%%%%%%%%%%%%%%%%%%%%%%%%%%%%%%%%%%%%%%%%%%%%%%%%%%%%%%%%%%%%%%%%%%%%%
%STATE 5: OPERATING
%%%%%%%%%%%%%%%%%%%%%%%%%%%%%%%%%%%%%%%%%%%%%%%%%%%%%%%%%%%%%%%%%%%%%%%%%%%

case 5

%Outputs for the state
PWMOnGrid               = 1;
CONNECT_GRID_CONTACT    = 1;
CONNECT_PRELOAD_CONTACT = 0;
selReactiveVoltageController = SEL_QVCONTROL;
initPLLGrid             = 1;
initReactiveVoltageController = 1;
initCurrentControllerG  = 1;
initDCControllerGrid    = 1;

%Counter initialisation
CONT_PRECHARGE   = 0;
CONT_CONNECT     = 0;
CONT_INIT_CC     = 0;

%Conditions to change state
if (CONNECT == 0)  %If connect equals zero
    state = 1;     %Dischonnect
end

%%%%%%%%%%%%%%%%%%%%%%%%%%%%%%%%%%%%%%%%%%%%%%%%%%%%%%%%%%%%%%%%%%%%%%%%%%%
%STATE MACHINE: END STATE MACHINE
%%%%%%%%%%%%%%%%%%%%%%%%%%%%%%%%%%%%%%%%%%%%%%%%%%%%%%%%%%%%%%%%%%%%%%%%%%%

end 

%%%%%%%%%%%%%%%%%%%%%%%%%%%%%%%%%%%%%%%%%%%%%%%%%%%%%%%%%%%%%%%%%%%%%%%%%%%
%INCREASE AND RESET COUNTERS
%%%%%%%%%%%%%%%%%%%%%%%%%%%%%%%%%%%%%%%%%%%%%%%%%%%%%%%%%%%%%%%%%%%%%%%%%%%

%PRECHARGE counter
if (CONT_PRECHARGE == 1)
    CONT_PRECHARGE = CONT_PRECHARGE_ANT + CONT_PRECHARGE;
else
    CONT_PRECHARGE = 0;
end

%CONNECT counter
if (CONT_CONNECT == 1)
    CONT_CONNECT = CONT_CONNECT_ANT + CONT_CONNECT;
else
    CONT_CONNECT = 0;
end

%INIT_CC counter
if (CONT_INIT_CC == 1)
    CONT_INIT_CC = CONT_INIT_CC_ANT + CONT_INIT_CC;
else
    CONT_INIT_CC = 0;
end

%%%%%%%%%%%%%%%%%%%%%%%%%%%%%%%%%%%%%%%%%%%%%%%%%%%%%%%%%%%%%%%%%%%%%%%%%%%
%OUTPUT GENERATOR
%%%%%%%%%%%%%%%%%%%%%%%%%%%%%%%%%%%%%%%%%%%%%%%%%%%%%%%%%%%%%%%%%%%%%%%%%%%

%Vector of outputs
outputs = [PWMOnGrid CONNECT_GRID_CONTACT CONNECT_PRELOAD_CONTACT selReactiveVoltageController initPLLGrid initReactiveVoltageController initCurrentControllerG initDCControllerGrid]';

%Vector of outputs
nowState = state;

%Vector with new counters
nowCounters = [CONT_PRECHARGE CONT_CONNECT CONT_INIT_CC]';

== matlab function B2B_2x15kW_LCO_paralelo_y_serie/VSC1 Controller2/dq to abc/udq Limitation ==
  settings: fimath=|
      | fimath(...
      | 'RoundMode', 'floor',...
      | 'OverflowMode', 'wrap',...
      | 'ProductMode', 'KeepLSB', 'ProductWordLength', 32,...
      | 'SumMode', 'KeepLSB', 'SumWordLength', 32,...
      | 'CastBeforeSum', false)
  data: vscG_ugdqRef input size=2; vscG_egdqPos input; vscG_ugdqSat output size=2; WNG_L12_IMAXG input
%Name: Saturation of the reference voltage inside the unit circle
%Developed: Emilio Bueno
%Modified: Javier Roldan

function vscG_ugdqSat = fcn(vscG_ugdqRef, vscG_egdqPos, WNG_L12_IMAXG)

%Definition of the inputs
ud_c = vscG_ugdqRef(1);
uq_c = vscG_ugdqRef(2);
WN_G = WNG_L12_IMAXG(1);
L12 = WNG_L12_IMAXG(2);
I_MAX_G = WNG_L12_IMAXG(3);

%Initialisation of the outputs
vscG_ugdqSat = [0 0]';

%We obtain the modulus
edq = sqrt(vscG_egdqPos(1)^2+vscG_egdqPos(2)^2)*(sqrt(2/3)); %Invariant power transformation, sqrt(2/3)

%Calculation of the maximum values
I_MAX_G_PEAK = I_MAX_G*sqrt(2);          %Maximum peak value
udqmax       = edq+WN_G*L12*I_MAX_G_PEAK;  %Maximum reachable voltage
udqmin       = edq-WN_G*L12*I_MAX_G_PEAK;  %Minimum reachable voltage

%We obtain the angle
theta = atan2(uq_c, ud_c);

%Saturation of the output
if ((ud_c*ud_c)+(uq_c*uq_c)) > (udqmax*udqmax*sqrt(2)) %Ouside the circle
    %vscG_ugdqSat(1) = udqmax*cos(theta);
    %vscG_ugdqSat(2) = udqmax*sin(theta); 
    vscG_ugdqSat(1) = ud_c;
    vscG_ugdqSat(2) = uq_c;
elseif ((ud_c*ud_c)+(uq_c*uq_c)) < (udqmin*udqmin*sqrt(2)) %Outside the circle
    %vscG_ugdqSat(1) = udqmin*cos(theta); 
    %vscG_ugdqSat(2) = udqmin*sin(theta);
    vscG_ugdqSat(1) = ud_c;
    vscG_ugdqSat(2) = uq_c;
else    %With no constraint
    vscG_ugdqSat(1) = ud_c;
    vscG_ugdqSat(2) = uq_c;
end

== matlab function B2B_2x15kW_LCO_paralelo_y_serie/VSC1 Controller2/Grid Side Measurements/D-LCO FLL/Sequence Detection/LCO_FLL_2_harm_alfa1/LCO_FLL_01 ==
  settings: fimath=|
      | fimath(...
      | 'RoundMode', 'floor',...
      | 'OverflowMode', 'wrap',...
      | 'ProductMode', 'KeepLSB', 'ProductWordLength', 32,...
      | 'SumMode', 'KeepLSB', 'SumWordLength', 32,...
      | 'CastBeforeSum', false)
  data: x1 input; x1p output; x2 input; x3 input; A input; v input; x2p output; x3p output; w output; k input
function [x1p,x2p,x3p,w] = fcn(x1, x2, x3, A, v, k)

%16/11/2021
%LCO-FLL for around 50Hz
%By Erick Israel Vázquez Oviedo
% Constants
wffw = 2*pi*235; %Initial frequency 
%k = 0.1; a controlar
gama = 1;
w = x3 + wffw;
ev = v - x2; % Error between reference and x2 to synchronize

% Diferential equations
x1p = (           (x1) + (x2) - ((1/(A*A))*x1*((x1*x1)+(x2*x2)))  )*w;
x2p = ( (k*ev) + (-x1) + (x2) - ((1/(A*A))*x2*((x1*x1)+(x2*x2)))  )*w;
x3p = -gama*ev*x1; % x1 is in quadrature with x2, 90 degrees delay

== matlab function B2B_2x15kW_LCO_paralelo_y_serie/VSC1 Controller2/Grid Side Measurements/D-LCO FLL/Sequence Detection/LCO_FLL_2_harm_alfa/LCO_FLL_01 ==
  settings: fimath=|
      | fimath(...
      | 'RoundMode', 'floor',...
      | 'OverflowMode', 'wrap',...
      | 'ProductMode', 'KeepLSB', 'ProductWordLength', 32,...
      | 'SumMode', 'KeepLSB', 'SumWordLength', 32,...
      | 'CastBeforeSum', false)
  data: x1 input; x1p output; x2 input; x3 input; A input; v input; x2p output; x3p output; w output; k input
function [x1p,x2p,x3p,w] = fcn(x1, x2, x3, A, v, k)

%16/11/2021
%LCO-FLL for around 50Hz
%By Erick Israel Vázquez Oviedo
% Constants
wffw = 2*pi*235; %Initial frequency 
%k = 2; a controlar
gama = 1;
w = x3 + wffw;
ev = v - x2; % Error between reference and x2 to synchronize

% Diferential equations
x1p = (           (x1) + (x2) - ((1/(A*A))*x1*((x1*x1)+(x2*x2)))  )*w;
x2p = ( (k*ev) + (-x1) + (x2) - ((1/(A*A))*x2*((x1*x1)+(x2*x2)))  )*w;
x3p = -gama*ev*x1; % x1 is in quadrature with x2, 90 degrees delay

== matlab function B2B_2x15kW_LCO_paralelo_y_serie/VSC1 Controller2/Grid Side Measurements/D-LCO FLL/Sequence Detection/LCO_FLL_3_harm_alfa/LCO_FLL_01 ==
  settings: fimath=|
      | fimath(...
      | 'RoundMode', 'floor',...
      | 'OverflowMode', 'wrap',...
      | 'ProductMode', 'KeepLSB', 'ProductWordLength', 32,...
      | 'SumMode', 'KeepLSB', 'SumWordLength', 32,...
      | 'CastBeforeSum', false)
  data: x1 input; x1p output; x2 input; x3 input; A input; v input; x2p output; x3p output; w output; k input
function [x1p,x2p,x3p,w] = fcn(x1, x2, x3, A, v, k)

%16/11/2021
%LCO-FLL for around 50Hz
%By Erick Israel Vázquez Oviedo
% Constants
wffw = 2*pi*550; %Initial frequency 
%k = 2; a controlar
gama = 1;
w = x3 + wffw;
ev = v - x2; % Error between reference and x2 to synchronize

% Diferential equations
x1p = (           (x1) + (x2) - ((1/(A*A))*x1*((x1*x1)+(x2*x2)))  )*w;
x2p = ( (k*ev) + (-x1) + (x2) - ((1/(A*A))*x2*((x1*x1)+(x2*x2)))  )*w;
x3p = -gama*ev*x1; % x1 is in quadrature with x2, 90 degrees delay

== matlab function B2B_2x15kW_LCO_paralelo_y_serie/VSC2 Controller/Grid Side Measurements/DSOGI QSG PLL/Sequence Detection/Sequence Detection ==
  settings: fimath=|
      | fimath(...
      | 'RoundMode', 'floor',...
      | 'OverflowMode', 'wrap',...
      | 'ProductMode', 'KeepLSB', 'ProductWordLength', 32,...
      | 'SumMode', 'KeepLSB', 'SumWordLength', 32,...
      | 'CastBeforeSum', false)
  data: ealphapos input; input_pll output; secuencia output; ebetapos input; ealphaneg input; ebetaneg input; theta input; edpos output; eqpos output; edneg output; eqneg output
function [input_pll, secuencia, edpos, eqpos, edneg, eqneg] = fcn(ealphapos, ebetapos, ealphaneg, ebetaneg, theta)

%Computation of negative and positive sequence module
module_ealphabetapos = sqrt(ealphapos^2+ebetapos^2);
module_ealphabetaneg = sqrt(ealphaneg^2+ebetaneg^2);

%Sequence detection
if (module_ealphabetapos >= module_ealphabetaneg)
    secuencia = +1; %Positive sequence
else
    secuencia = -1; %Negative sequence
end

%Positive sequence calculation
edpos = ealphapos*cos(theta)+ebetapos*sin(theta);
eqpos = -ealphapos*sin(theta)+ebetapos*cos(theta);

%Negative sequence calculation
edneg = ealphaneg*cos(theta)-ebetaneg*sin(theta);
eqneg = ealphaneg*sin(theta)+ebetaneg*cos(theta);

%Output calculation
if (secuencia == 1)
    eqpos_pu = eqpos/module_ealphabetapos;
    input_pll = eqpos_pu;
else 
    eqneg_pu = eqneg/module_ealphabetaneg;
    input_pll = eqneg_pu;
end
